simulink model "Control_systemR2024a"  (R2025b)
settings: Solver=FixedStepAuto  StartTime=0.0  StopTime=10  FixedStep=0.01  RelTol=1e-3
values from neighbouring files (symbols this model uses):
  beta = beta(:)    [MCN2.m]    (also in initialize_s_bow.m = [beta1,beta2]; rounded_step_gen.m = -alpha*t1*t1; untitled.m = [beta1; beta2])
  calMp = Adgsl10m1'*calM1*Adgsl10m1    [initialize_s_bow.m]    (also in untitled.m = zeros(6,6,2))
  lM = zeros(2)    [initialize_s_bow.m]    (also in untitled.m = zeros(n,n))
  xi = [xi1,xi2]    [initialize_s_bow.m]    (also in untitled.m = [xi1, xi2])
settings Model: Creator=81135  LastModifiedBy=dixiao

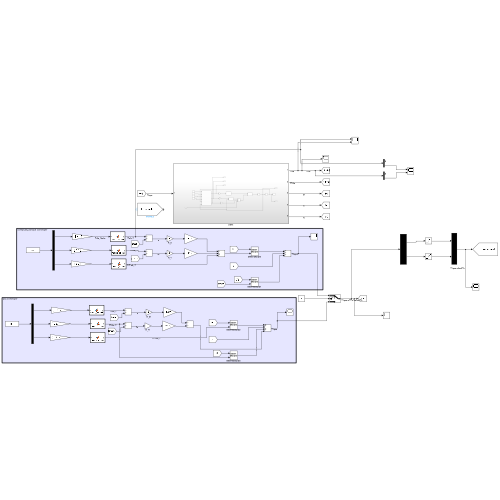
[thumbnail: Simulink's stored preview of the top-level diagram]
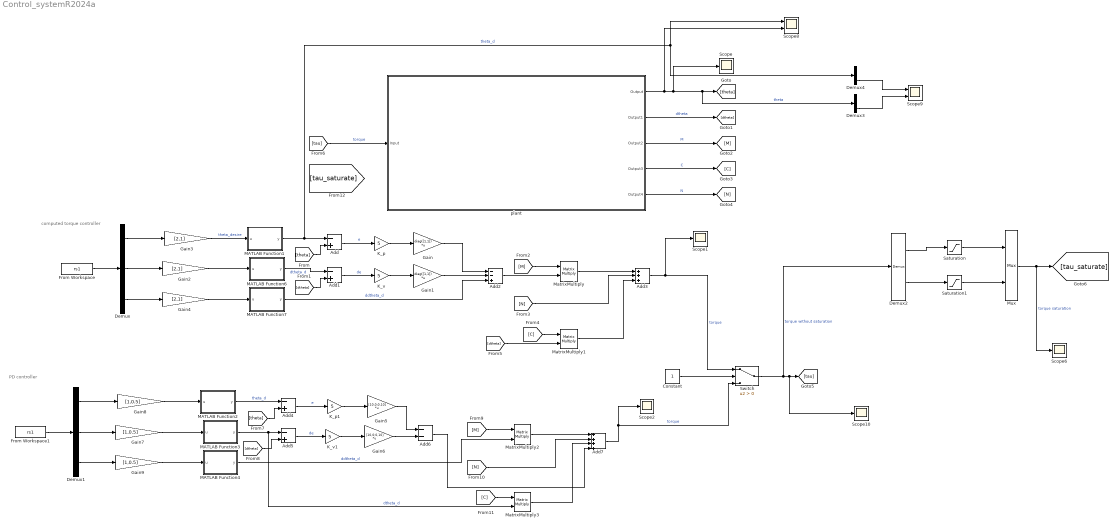
== system Control_systemR2024a ==
  note: PD controller
  note: computed torque controller
  Add{,1,4..5} (4 alike) : Sum  Inputs=-+
  Add2 : Sum  Inputs=--+
  Add3 : Sum  Inputs=+++
  Add6 : Sum  Inputs=--
  Add7 : Sum  Inputs=++++
  Constant : Constant
  Demux : Demux  Outputs=3
  Demux1 : Demux  Outputs=3
  Demux2 : Demux  Outputs=2
  Demux3 : Demux  Outputs=2
  Demux4 : Demux  Outputs=2
  From Workspace : FromWorkspace  VariableName=rs1
  From Workspace1 : FromWorkspace  VariableName=rs1
  Gain : Gain  Gain=diag([1,1])  Multiplication=Matrix(K*u)
  Gain1 : Gain  Gain=diag([1,1])  Multiplication=Matrix(K*u)
  Gain2 : Gain  Gain=[2,1]
  Gain3 : Gain  Gain=[2,1]
  Gain4 : Gain  Gain=[2,1]
  Gain5 : Gain  Gain=[10,0;0,10]  Multiplication=Matrix(K*u)
  Gain6 : Gain  Gain=[10,0;0,10]  Multiplication=Matrix(K*u)
  Gain7 : Gain  Gain=[1,0.5]
  Gain8 : Gain  Gain=[1,0.5]
  Gain9 : Gain  Gain=[1,0.5]
  K_p : Gain  Gain=5
  K_p1 : Gain  Gain=5
  K_v : Gain  Gain=5
  K_v1 : Gain  Gain=5
  MATLAB Function1 : MATLAB Function  TreatAsAtomicUnit=on
  MATLAB Function2 : MATLAB Function  TreatAsAtomicUnit=on
  MATLAB Function3 : MATLAB Function  TreatAsAtomicUnit=on
  MATLAB Function4 : MATLAB Function  TreatAsAtomicUnit=on
  MATLAB Function6 : MATLAB Function  TreatAsAtomicUnit=on
  MATLAB Function7 : MATLAB Function  TreatAsAtomicUnit=on
  MatrixMultiply{,1..3} (4 alike) : Product  Multiplication=Matrix(*)
  Mux : Mux  Inputs=2
  Saturation : Saturate  UpperLimit=200  LowerLimit=-100
  Saturation1 : Saturate  UpperLimit=1000  LowerLimit=-1000
  Scope{,1..2,6,10} (5 alike) : Scope
      Scope settings: ActiveDisplayYMinimum=-0.1296  ActiveDisplayYMaximum=1.16638
      Scope1 settings: ActiveDisplayYMinimum=-1  ActiveDisplayYMaximum=1  DataLoggingVariableName=ScopeData3
      Scope10 settings: ActiveDisplayYMinimum=-1  ActiveDisplayYMaximum=1  DataLoggingVariableName=ScopeData4
      Scope2 settings: ActiveDisplayYMinimum=-5091.129  ActiveDisplayYMaximum=5351.713  DataLoggingVariableName=ScopeData2
      Scope6 settings: ActiveDisplayYMinimum=-1  ActiveDisplayYMaximum=1  DataLoggingVariableName=ScopeData7
  Scope8 : Scope  NumInputPorts=2
      settings: ActiveDisplayYMinimum=-0.25041687770145205  ActiveDisplayYMaximum=2.2537518993130687  DataLoggingVariableName=ScopeData2
  Scope9 : Scope  NumInputPorts=2
      settings: ActiveDisplayYMinimum=-0.12501577875372782  ActiveDisplayYMaximum=1.1251420087835506  DataLoggingVariableName=ScopeData3
  Switch : Switch  Criteria=u2 > Threshold  SaturateOnIntegerOverflow=off  InputSameDT=off
  plant : Subsystem
  wires:
  plant/1(Output) -> Scope8/2, Demux3/1, [theta], Scope/1  "theta"
  plant/2(Output1) -> [dtheta]  "dtheta"
  plant/3(Output2) -> [M]  "M"
  plant/4(Output3) -> [C]  "C"
  plant/5(Output4) -> [N]  "N"
  Add/1 -> K_p/1  "e"
  [dtheta] -> MatrixMultiply1/2
  MatrixMultiply/1 -> Add3/1
  Gain1/1 -> Add2/2
  Demux/2 -> Gain2/1
  [N] -> Add3/2
  From Workspace/1 -> Demux/1
  [theta] -> Add/2
  Add1/1 -> K_v/1  "de"
  MATLAB Function6/1(y) -> Add1/1  "dtheta_d"
  [M] -> MatrixMultiply/1
  [dtheta] -> Add1/2
  Add3/1 -> Switch/1, Scope1/1  "torque"
  [C] -> MatrixMultiply1/1
  Add2/1 -> MatrixMultiply/2
  MATLAB Function7/1(y) -> Add2/3  "ddtheta_d"
  MatrixMultiply1/1 -> Add3/3
  Gain/1 -> Add2/1
  Demux/1 -> Gain3/1
  MATLAB Function1/1(y) -> Demux4/1, Scope8/1, Add/1  "theta_d"
  Gain4/1 -> MATLAB Function7/1(u)
  Gain2/1 -> MATLAB Function6/1(u)
  Gain3/1 -> MATLAB Function1/1(u)  "theta_desire"
  K_v/1 -> Gain1/1
  K_p/1 -> Gain/1
  Demux/3 -> Gain4/1
  [N] -> Add7/2
  Demux1/2 -> Gain7/1
  Gain6/1 -> Add6/2
  Add4/1 -> K_p1/1  "e"
  [C] -> MatrixMultiply3/1
  Add7/1 -> Switch/3, Scope2/1  "torque"
  MatrixMultiply3/1 -> Add7/3
  Gain5/1 -> Add6/1
  MATLAB Function4/1(y) -> MatrixMultiply2/2  "ddtheta_d"
  Demux1/1 -> Gain8/1
  Gain9/1 -> MATLAB Function4/1(u)
  Gain8/1 -> MATLAB Function2/1(u)
  Gain7/1 -> MATLAB Function3/1(u)
  MATLAB Function2/1(y) -> Add4/1  "theta_d"
  From Workspace1/1 -> Demux1/1
  MatrixMultiply2/1 -> Add7/1
  Demux1/3 -> Gain9/1
  K_v1/1 -> Gain6/1
  [M] -> MatrixMultiply2/1
  MATLAB Function3/1(y) -> MatrixMultiply3/2, Add5/1  "dtheta_d"
  [dtheta] -> Add5/2
  Add5/1 -> K_v1/1  "de"
  K_p1/1 -> Gain5/1
  [theta] -> Add4/2
  Add6/1 -> Add7/4
  Constant/1 -> Switch/2
  Demux2/2 -> Saturation1/1
  Demux2/1 -> Saturation/1
  Switch/1 -> Demux2/1, Scope10/1, [tau]  "torque without saturation"
  Saturation/1 -> Mux/1
  Saturation1/1 -> Mux/2
  Mux/1 -> Scope6/1, [tau_saturate]  "torque saturation"
  Demux4/2 -> Scope9/1
  Demux3/2 -> Scope9/2
  [tau] -> plant/1(Input)  "torque"

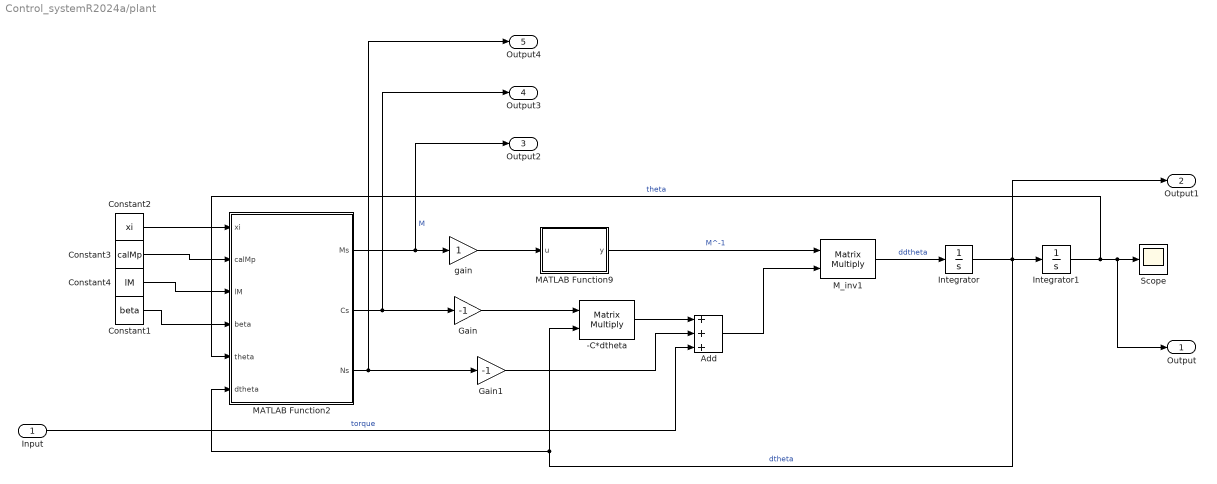
== system Control_systemR2024a/plant ==
  Input : Inport
  -C*dtheta : Product  Multiplication=Matrix(*)
  Add : Sum  Inputs=+++
  Constant1 : Constant  Value=beta
  Constant2 : Constant  Value=xi
  Constant3 : Constant  Value=calMp
  Constant4 : Constant  Value=lM
  Gain : Gain  Gain=-1
  Gain1 : Gain  Gain=-1
  Integrator : Integrator  InitialCondition=[0;0]
  Integrator1 : Integrator  InitialCondition=[0;0]
  MATLAB Function2 : MATLAB Function  TreatAsAtomicUnit=on
  MATLAB Function9 : MATLAB Function  TreatAsAtomicUnit=on
  M_inv1 : Product  Multiplication=Matrix(*)
  Scope : Scope
      settings: ActiveDisplayYMinimum=-0.1296  ActiveDisplayYMaximum=1.16638
  gain : Gain
  Output : Outport
  Output1 : Outport  Port=2
  Output2 : Outport  Port=3
  Output3 : Outport  Port=4
  Output4 : Outport  Port=5
  wires:
  MATLAB Function2/1(Ms) -> Output2/1, gain/1  "M"
  Integrator/1 -> Output1/1, -C*dtheta/2, MATLAB Function2/6(dtheta), Integrator1/1  "dtheta"
  Gain/1 -> -C*dtheta/1
  Constant4/1 -> MATLAB Function2/3(lM)
  -C*dtheta/1 -> Add/1
  Constant3/1 -> MATLAB Function2/2(calMp)
  Integrator1/1 -> MATLAB Function2/5(theta), Output/1, Scope/1  "theta"
  M_inv1/1 -> Integrator/1  "ddtheta"
  MATLAB Function2/3(Ns) -> Output4/1, Gain1/1
  Constant1/1 -> MATLAB Function2/4(beta)
  Gain1/1 -> Add/2
  gain/1 -> MATLAB Function9/1(u)
  MATLAB Function2/2(Cs) -> Output3/1, Gain/1
  Constant2/1 -> MATLAB Function2/1(xi)
  Add/1 -> M_inv1/2
  MATLAB Function9/1(y) -> M_inv1/1  "M^-1"
  Input/1 -> Add/3  "torque"

== matlab function Control_systemR2024a/MATLAB Function2 ==
  data: u input; y output
function y = matrix_column(u)

    y = u(:);
end

== matlab function Control_systemR2024a/plant/MATLAB Function2 ==
  data: xi input; Ms output; calMp input; lM input; beta input; theta input; dtheta input; Cs output; Ns output
function [Ms,Cs,Ns] = MCNsim(xi,calMp,lM,beta,theta,dtheta)
    n = length(theta);
    Ms = zeros(n, n);
    Cs = zeros(n, n);
    % Ns = zeros(n, 1);
    
    % ========== 关键步骤1：预先计算所有需要的变换矩阵 g = exp(ξθ) ==========
    g = cell(1, n+1);
    g{1} = eye(4);
    for i = 1:n
        xi_i = xi(:, i);
        g_joint = expm(hat_se3(xi_i) * theta(i));
        g{i+1} = g{i} * g_joint;
    end
    
    % ========== 关键步骤2：计算所有 A_{ij} ==========
    A = cell(n, n);
    for i = 1:n
        for j = 1:n
            if i > j
                g_ji = inv(g{j+1}) * g{i+1};
                A{i,j} = inv(adjmg(g_ji));
            elseif i == j
                A{i,j} = eye(6);
            else
                A{i,j} = zeros(6);
            end
        end
    end
    
    % ========== 步骤3：计算惯性矩阵 M ==========
    for i = 1:n
        for j = 1:n
            M_ij = 0;
            for l = lM(i, j):n
                M_l = calMp(1:6, 1:6, l);
                term = xi(:, i)' * A{l, i}' * M_l * A{l, j} * xi(:, j);
                M_ij = M_ij + term;
            end
            Ms(i, j) = M_ij;
        end
    end
    
    % ========== 步骤4：计算科氏矩阵 C（解析公式） ==========
    for i = 1:n
        for j = 1:n
            C_ij = 0;
            for k = 1:n
                dM_ij_dtheta_k = compute_partial_M(xi, calMp, lM, A, i, j, k, n);
                dM_ik_dtheta_j = compute_partial_M(xi, calMp, lM, A, i, k, j, n);
                dM_kj_dtheta_i = compute_partial_M(xi, calMp, lM, A, k, j, i, n);
                C_ij = C_ij + 0.5 * (dM_ij_dtheta_k + dM_ik_dtheta_j - dM_kj_dtheta_i) * dtheta(k);
            end
            Cs(i, j) = C_ij;
        end
    end
    
    % ========== 步骤5：计算 N（根据图片公式和你的物理参数） ==========
    % 定义物理参数（与主脚本保持一致）
    r1 = 0.36;      % 0.9 * 0.4
    r2 = 0.315;     % 0.7 * 0.45
    g_val = 9.81;
    m1 = 35;
    m2 = 25;
    l1 = 0.9;

    % 计算势能梯度 ∂V/∂θ（解析式，无需符号）
    th1 = theta(1);
    th2 = theta(2);
    grad_V = zeros(n,1);
    grad_V(1) = m1*g_val*r1*sin(th1) + m2*g_val*(l1*sin(th1) + r2*sin(th1+th2));
    grad_V(2) = m2*g_val*r2*sin(th1+th2);

    % 摩擦项
    friction_term = beta(:) .* dtheta(:);

    % 最终 Ns（因为你的方程是 tau = M*ddq + C*dq + Ns）
    Ns = grad_V + friction_term;
end

% ========== 辅助函数：计算重力势能梯度 ∂V/∂θ (已根据你的代码调整) ==========


% ========== 其他辅助函数保持不变 ==========
function dM_ij_dtheta_k = compute_partial_M(xi, calMp, lM, A, i, j, k, n)
    dM_ij_dtheta_k = 0;
    
    for l = lM(i, j):n
        M_l = calMp(1:6, 1:6, l);
        xi_i = xi(:, i);
        xi_j = xi(:, j);
        xi_k = xi(:, k);
        
        if k <= l
            % 计算 ad(A_{ki} * xi_i)
            A_ki_xi_i = A{k, i} * xi_i;
            ad_Aki_xi_i = adjoint_lie_algebra(A_ki_xi_i);
            
            % 计算 ad(A_{kj} * xi_j)
            A_kj_xi_j = A{k, j} * xi_j;
            ad_Akj_xi_j = adjoint_lie_algebra(A_kj_xi_j);
            
            term1 = (ad_Aki_xi_i * xi_k)' * A{l, k}' * M_l * A{l, j} * xi_j;
            term2 = xi_i' * A{l, i}' * M_l * A{l, k} * (ad_Akj_xi_j * xi_k);
            
            dM_ij_dtheta_k = dM_ij_dtheta_k + term1 + term2;
        end
    end
end

function ad_xi = adjoint_lie_algebra(xi)
    v = xi(1:3);
    w = xi(4:6);
    w_hat = hatm_num(w);
    v_hat = hatm_num(v);
    ad_xi = [w_hat, v_hat;
             zeros(3), w_hat];
end

function se3 = hat_se3(xi)
    v = xi(1:3);
    w = xi(4:6);
    se3 = [hatm_num(w), v;
           zeros(1,3), 0];
end

== matlab function Control_systemR2024a/MATLAB Function1 ==
  data: u input; y output
function y = matrix_column(u)

    y = u(:);
end

== matlab function Control_systemR2024a/MATLAB Function6 ==
  data: u input; y output
function y = matrix_column(u)

    y = u(:);
end

== matlab function Control_systemR2024a/MATLAB Function7 ==
  data: u input; y output
function y= matrix_column(u)

    y = u(:);
end

== matlab function Control_systemR2024a/MATLAB Function3 ==
  data: u input; y output
function y = matrix_column(u)

    y = u(:);
end

== matlab function Control_systemR2024a/MATLAB Function4 ==
  data: u input; y output
function y= matrix_column(u)

    y = u(:);
end

== matlab function Control_systemR2024a/plant/MATLAB Function9 ==
  data: u input; y output
function y = matrix_inv(u)

    y = inv(u);
end
